simulink model "MIT_SIN_NORMALIZAR"  (Simulink 5.0)
settings: Solver=ode45  StartTime=0.0  StopTime=500  FixedStep=6  RelTol=1e-3
undefined symbols (not defined in the file): a1, a2, am, Gama, Km
settings Model: LastModifiedBy=Administrador  RTWOptions="-aEnforceIntegerDowncast=1 -aExtMode=0 -aExtModeTesting=0 -aFoldNonRolledExpr=1 -aForceParamTrailComments=0 -aGenerateComments=1 -aGenerateReport=0 -aIgnoreCustomStorageClasses=1 -aIncDataTypeInIds=0 -aIncHierarchyInIds=0 -aInlineInvariantSignals=0 -aInlinedPrmAccess=\"Literals\" -aLocalBlockOutputs=1 -aLogVarNameModifier=\"rt_\" -aMaxRTWIdLen=31 -aPrefixModelToSubsysFcnNames=1 -aRTWVerbose=1 -aRollThreshold=5 -aShowEliminatedStatements=0"

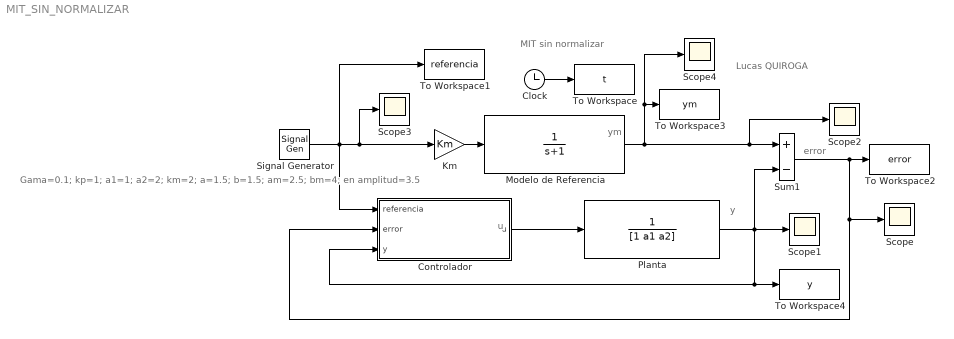
== system MIT_SIN_NORMALIZAR ==
  note: y
  note: ym
  note: u
  note: error
  note: MIT sin normalizar
  note: Lucas QUIROGA
  note: Gama=0.1;
      | kp=1;
      | a1=1;
      | a2=2;
      | km=2;
      | a=1.5;
      | b=1.5;
      | am=2.5;
      | bm=4;
      | en amplitud=3.5
  Clock : Clock
  Controlador : Subsystem
  Km : Gain  Gain=Km  SaturateOnIntegerOverflow=on
  Modelo de Referencia : TransferFcn  Denominator=[1 1]
  Planta : TransferFcn  Denominator=[1 a1 a2]
  Scope{,1..4} (5 alike) : Scope
      Scope2 settings: SaveName=ScopeData2
      Scope3 settings: SaveName=ScopeData3
      Scope4 settings: SaveName=ScopeData6
  Signal Generator : SignalGenerator  WaveForm=square  Amplitude=3.5  Frequency=0.05
  Sum1 : Sum  Inputs=+-  SaturateOnIntegerOverflow=on
  To Workspace : ToWorkspace  VariableName=t  SampleTime=-1  SaveFormat=Array
  To Workspace1 : ToWorkspace  VariableName=referencia  SampleTime=-1  SaveFormat=Array
  To Workspace2 : ToWorkspace  VariableName=error  SampleTime=-1  SaveFormat=Array
  To Workspace3 : ToWorkspace  VariableName=ym  SampleTime=-1  SaveFormat=Array
  To Workspace4 : ToWorkspace  VariableName=y  SampleTime=-1  SaveFormat=Array
  wires:
  Controlador/1(u) -> Planta/1
  Signal Generator/1 -> Controlador/1(referencia), To Workspace1/1, Scope3/1, Km/1
  Modelo de Referencia/1 -> Sum1/1, Scope2/1, To Workspace3/1, Scope4/1
  Sum1/1 -> To Workspace2/1, Controlador/2(error), Scope/1
  Clock/1 -> To Workspace/1
  Planta/1 -> Sum1/2, Scope1/1, To Workspace4/1, Controlador/3(y)
  Km/1 -> Modelo de Referencia/1

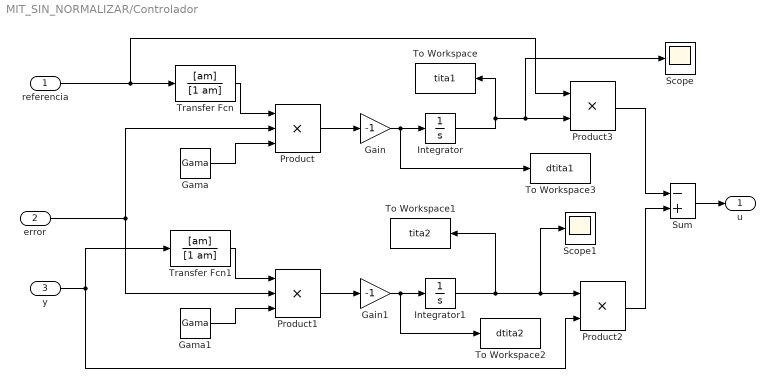
== system MIT_SIN_NORMALIZAR/Controlador ==
  referencia : Inport
  error : Inport  Port=2
  y : Inport  Port=3
  Gain : Gain  Gain=-1  SaturateOnIntegerOverflow=on
  Gain1 : Gain  Gain=-1  SaturateOnIntegerOverflow=on
  Gama : Constant  Value=Gama
  Gama1 : Constant  Value=Gama
  Integrator : Integrator
  Integrator1 : Integrator
  Product : Product  Inputs=3  SaturateOnIntegerOverflow=on
  Product1 : Product  Inputs=3  SaturateOnIntegerOverflow=on
  Product2 : Product  SaturateOnIntegerOverflow=on
  Product3 : Product  SaturateOnIntegerOverflow=on
  Scope : Scope
      settings: SaveName=ScopeData4
  Scope1 : Scope
      settings: SaveName=ScopeData5
  Sum : Sum  Inputs=-+  SaturateOnIntegerOverflow=on
  To Workspace : ToWorkspace  VariableName=tita1  SampleTime=-1  SaveFormat=Array
  To Workspace1 : ToWorkspace  VariableName=tita2  SampleTime=-1  SaveFormat=Array
  To Workspace2 : ToWorkspace  VariableName=dtita2  SampleTime=-1  SaveFormat=Array
  To Workspace3 : ToWorkspace  VariableName=dtita1  SampleTime=-1  SaveFormat=Array
  Transfer Fcn : TransferFcn  Numerator=[am]  Denominator=[1 am]
  Transfer Fcn1 : TransferFcn  Numerator=[am]  Denominator=[1 am]
  u : Outport
  wires:
  Gain/1 -> Integrator/1, To Workspace3/1
  Product/1 -> Gain/1
  Transfer Fcn/1 -> Product/1
  Gama/1 -> Product/3
  Integrator/1 -> To Workspace/1, Product3/2, Scope/1
  Gain1/1 -> Integrator1/1, To Workspace2/1
  Product1/1 -> Gain1/1
  Transfer Fcn1/1 -> Product1/1
  Gama1/1 -> Product1/3
  Integrator1/1 -> To Workspace1/1, Product2/1, Scope1/1
  referencia/1 -> Product3/1, Transfer Fcn/1
  error/1 -> Product1/2, Product/2
  y/1 -> Product2/2, Transfer Fcn1/1
  Product2/1 -> Sum/2
  Product3/1 -> Sum/1
  Sum/1 -> u/1
